simulink model "observer_lb"  (R2022b)
settings: Solver=VariableStepAuto  StartTime=0.0  StopTime=20.0  RelTol=1e-3
settings Model: Creator=integzz  LastModifiedBy=integzz

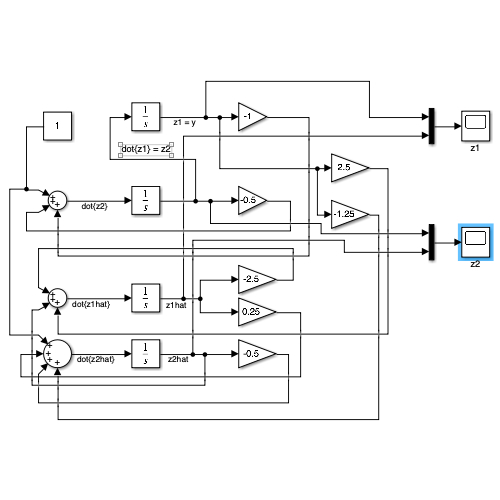
[thumbnail: Simulink's stored preview of the top-level diagram]
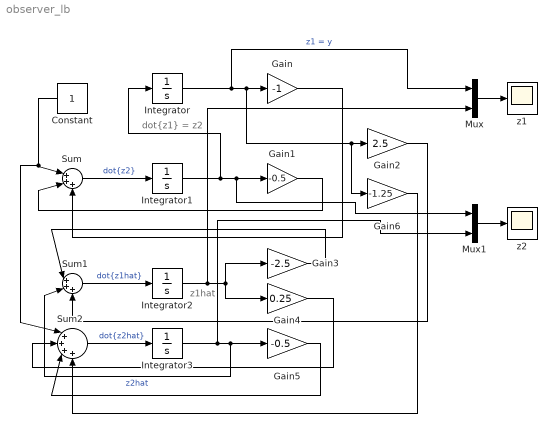
== system observer_lb ==
  note: z1hat
  note: dot{z1} = z2
  Constant : Constant
  Gain : Gain  Gain=-1
  Gain1 : Gain  Gain=-0.5
  Gain2 : Gain  Gain=2.5
  Gain3 : Gain  Gain=-2.5
  Gain4 : Gain  Gain=0.25
  Gain5 : Gain  Gain=-0.5
  Gain6 : Gain  Gain=-1.25
  Integrator : Integrator
  Integrator1 : Integrator
  Integrator2 : Integrator
  Integrator3 : Integrator  InitialCondition=1
  Mux : Mux  Inputs=2
  Mux1 : Mux  Inputs=2
  Sum : Sum  Inputs=|+++
  Sum1 : Sum  Inputs=|+++
  Sum2 : Sum  Inputs=|++++
  z1 : Scope
  z2 : Scope
  wires:
  Integrator1/1 -> Mux1/1, Gain1/1, Integrator/1
  Sum/1 -> Integrator1/1  "dot{z2}"
  Gain/1 -> Sum/3
  Gain1/1 -> Sum/2
  Integrator/1 -> Mux/1, Gain6/1, Gain2/1, Gain/1  "z1 = y"
  Constant/1 -> Sum2/1, Sum/1
  Sum1/1 -> Integrator2/1  "dot{z1hat}"
  Gain2/1 -> Sum1/3
  Integrator2/1 -> Mux/2, Gain4/1, Gain3/1
  Gain3/1 -> Sum1/1
  Integrator3/1 -> Mux1/2, Gain5/1, Sum1/2  "z2hat"
  Sum2/1 -> Integrator3/1  "dot{z2hat}"
  Gain4/1 -> Sum2/2
  Gain5/1 -> Sum2/3
  Gain6/1 -> Sum2/4
  Mux/1 -> z1/1
  Mux1/1 -> z2/1
